simulink model "motorVelocityControlSystem"  (R2017b)
settings: Solver=FixedStepAuto  StartTime=0.0  StopTime=Tend  RelTol=1e-3  EnableMultiTasking=on
PreLoadFcn:
  | params
InitFcn:
  | params
values from neighbouring files (symbols this model uses):
  Tend = 10    [params.m]
  Ts = 0.01    [params.m]
  Tstep = 5    [params.m]
libraries: arduinolib x4, cstblocks x1
settings Model: SimulationMode=external  ExtModeTrigDuration=2  Creator=s-tsujii  LastModifiedBy=s-tsujii
settings OptimizationCC: PassReuseOutputArgsThreshold=0  MaxStackSize=64
settings DebuggingCC: ParameterTunabilityLossMsg=error
settings HardwareCC: ProdBitPerInt=16  ProdBitPerPointer=16  ProdBitPerSizeT=16  ProdBitPerPtrDiffT=16  ProdLargestAtomicFloat=None  ProdWordSize=8  ProdHWDeviceType=Atmel->AVR  UseEmbeddedCoderFeatures=off  UseSimulinkCoderFeatures=off
settings SFSimCC: MATLABDynamicMemAlloc=off
settings RTWCC: SystemTargetFile=ert.tlc  HardwareBoard=Arduino Uno  TLCOptions=-aInlineSetEventsForThisBaseRateFcn=TLC_FALSE -aSuppressMultiTaskScheduler=TLC_FALSE -aRateBasedStepFcn=1  TemplateMakefile=ert_default_tmf  GenerateReport=on  Toolchain=Arduino AVR  BuildConfiguration=Faster Runs  LaunchReport=on
settings CodeAppCC: ForceParamTrailComments=on  OperatorAnnotations=on  MangleLength=10
settings ERTTargetCC: ERTCustomFileBanners=off  SupportContinuousTime=on  SupportNonInlinedSFcns=on  RemoveResetFunc=off  SupportVariableSizeSignals=on  ModelStepFunctionPrototypeControlCompliant=off

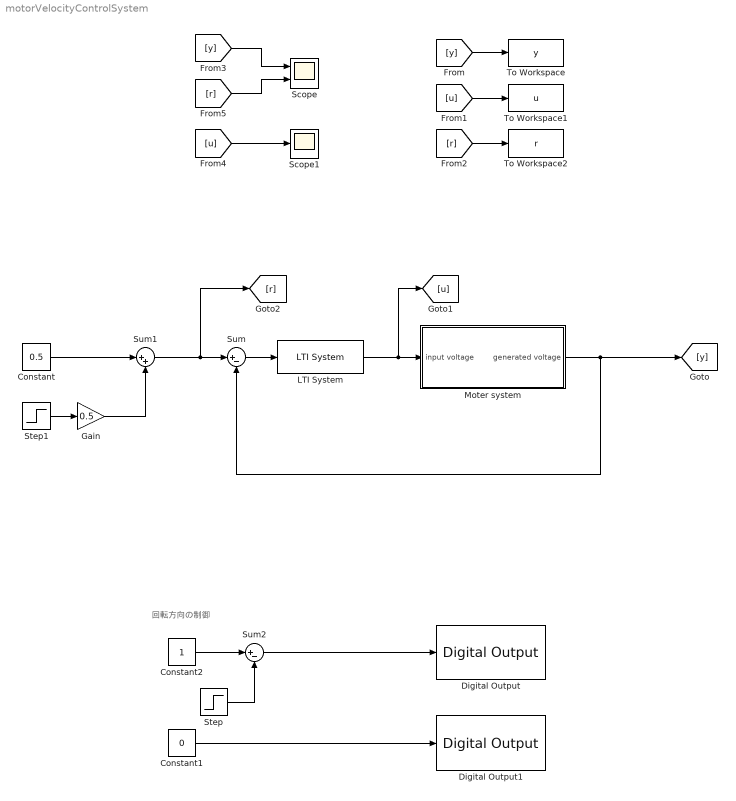
== system motorVelocityControlSystem ==
  note: 回転方向の制御
  Constant : Constant  Value=0.5
  Constant1 : Constant  Value=0
  Constant2 : Constant
  Digital Output : arduinolib/Digital Output  pinNumber=6  blockPlatform=arduino
  Digital Output1 : arduinolib/Digital Output  pinNumber=7  blockPlatform=arduino
  Gain : Gain  Gain=0.5
  LTI System : cstblocks/LTI System  sys=Cfb  IC=[]
  Moter system : Subsystem
  Scope : Scope  NumInputPorts=2
  Scope1 : Scope
  Step : Step  Time=Tend-Ts  SampleTime=Ts
  Step1 : Step  Time=Tstep  SampleTime=Ts
  Sum : Sum  Inputs=|+-
  Sum1 : Sum  Inputs=|++
  Sum2 : Sum  Inputs=|+-
  To Workspace : ToWorkspace  VariableName=y  SaveFormat=Structure With Time  SampleTime=-1
  To Workspace1 : ToWorkspace  VariableName=u  SaveFormat=Structure With Time  SampleTime=-1
  To Workspace2 : ToWorkspace  VariableName=r  SaveFormat=Structure With Time  SampleTime=-1
  wires:
  Sum/1 -> LTI System/1
  Sum1/1 -> [r], Sum/1
  Sum2/1 -> Digital Output/1
  Constant1/1 -> Digital Output1/1
  Constant2/1 -> Sum2/1
  Step/1 -> Sum2/2
  Moter system/1(generated voltage) -> Sum/2, [y]
  [y] -> To Workspace/1
  LTI System/1 -> [u], Moter system/1(input voltage)
  [u] -> To Workspace1/1
  [r] -> To Workspace2/1
  [y] -> Scope/1
  [r] -> Scope/2
  [u] -> Scope1/1
  Constant/1 -> Sum1/1
  Step1/1 -> Gain/1
  Gain/1 -> Sum1/2

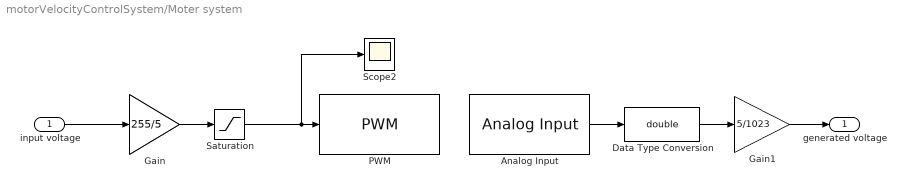
== system motorVelocityControlSystem/Moter system ==
  input voltage : Inport
  Analog Input : arduinolib/Analog Input  pinNumber=0  sampleTime=Ts  blockPlatform=arduino
  Data Type Conversion : DataTypeConversion  OutDataTypeStr=double
  Gain : Gain  Gain=255/5
  Gain1 : Gain  Gain=5/1023
  PWM : arduinolib/PWM  pinNumber=5  blockPlatform=arduino
  Saturation : Saturate  UpperLimit=255
  Scope2 : Scope
  generated voltage : Outport
  wires:
  Analog Input/1 -> Data Type Conversion/1
  Saturation/1 -> PWM/1, Scope2/1
  Gain1/1 -> generated voltage/1
  Data Type Conversion/1 -> Gain1/1
  input voltage/1 -> Gain/1
  Gain/1 -> Saturation/1
